simulink model "vtg"  (R2025b)
settings: Solver=FixedStepAuto  StartTime=0.0  StopTime=inf  FixedStep=0.05  RelTol=1e-3
libraries: robotlib x11
settings Model: Creator=sprinkle  LastModifiedBy=sprinkle
settings OptimizationCC: DefaultParameterBehavior=Inlined  EnhancedBackFolding=on  PassReuseOutputArgsAs=Individual arguments  ZeroExternalMemoryAtStartup=off  ZeroInternalMemoryAtStartup=off  MaxStackSize=64  OptimizeBlockOrder=speed  DifferentSizesBufferReuse=on  OptimizationCustomize=off  EfficientTunableParamExpr=on
settings DebuggingCC: ParameterTunabilityLossMsg=error
settings HardwareCC: ProdBitPerPointer=32.0  ProdBitPerSizeT=32.0  ProdBitPerPtrDiffT=32.0  ProdLargestAtomicFloat=None  ProdIntDivRoundTo=Undefined  ProdEndianess=Unspecified  ProdWordSize=32.0  ProdHWDeviceType=Generic->Unspecified (assume 32-bit Generic)
settings SFSimCC: MATLABDynamicMemAlloc=off
settings RTWCC: SystemTargetFile=ert.tlc  HardwareBoard=Robot Operating System (ROS)  TLCOptions="-aInlineSetEventsForThisBaseRateFcn=TLC_FALSE -aSuppressMultiTaskScheduler=TLC_FALSE  -aRateBasedStepFcn=0"  GenCodeOnly=on  TemplateMakefile=ert_default_tmf  Toolchain=Catkin  TargetLang=C++  Description=Embedded Coder
settings CodeAppCC: ForceParamTrailComments=on  IgnoreCustomStorageClasses=off  OperatorAnnotations=on  SimulinkDataObjDesc=on  SFDataObjDesc=on  InsertBlockDesc=on

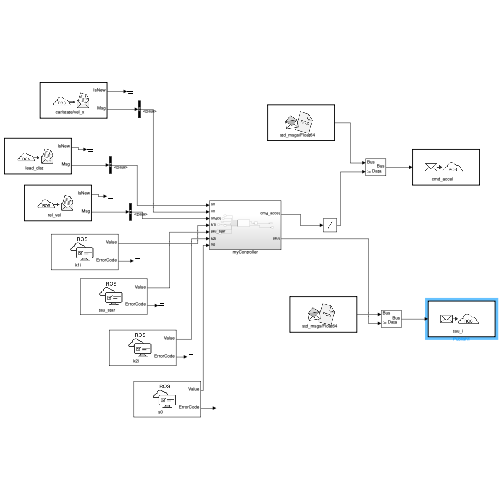
[thumbnail: Simulink's stored preview of the top-level diagram]
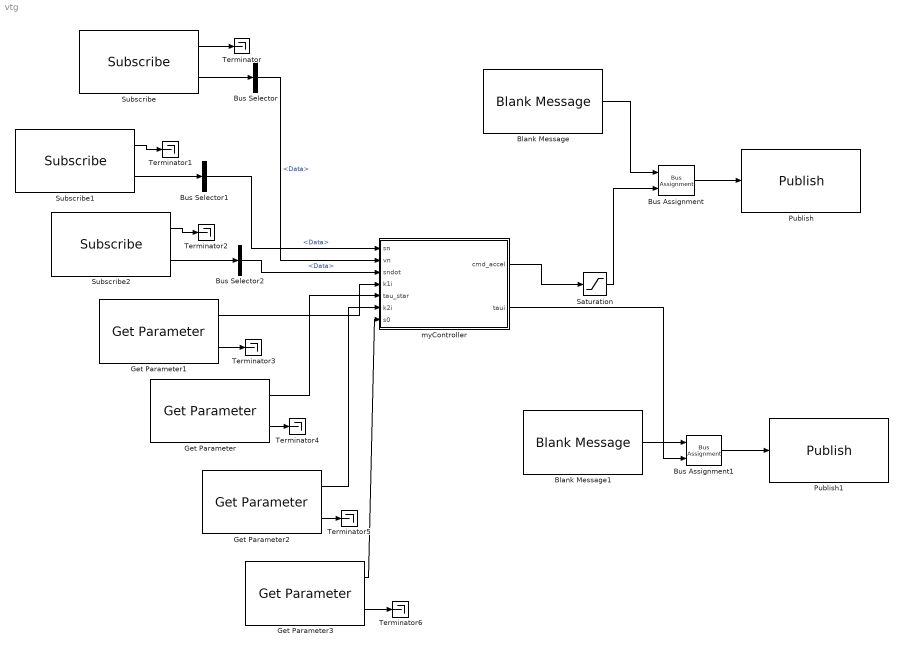
== system vtg ==
  Blank Message : robotlib/Blank Message  messageClass=Message  entityType=std_msgs/Float64  messageType=std_msgs/Float64  SampleTime=inf  legacyBusStruct=off
  Blank Message1 : robotlib/Blank Message  messageClass=Message  entityType=std_msgs/Float64  messageType=std_msgs/Float64  SampleTime=inf  legacyBusStruct=off
  Bus Assignment : BusAssignment  AssignedSignals=Data
  Bus Assignment1 : BusAssignment  AssignedSignals=Data
  Bus Selector : BusSelector  OutputSignals=Data
  Bus Selector1 : BusSelector  OutputSignals=Data
  Bus Selector2 : BusSelector  OutputSignals=Data
  Get Parameter : robotlib/Get Parameter  ParameterSource=Specify your own  ParameterName=tau_star  ParameterType=double  ParameterMaxArrayLength=16  ParameterInitialValue=2.0  SampleTime=-1  ShowErrorCodeOutput=on  ModelName=vtg  BlockId=ParamGet_vtg_18
  Get Parameter1 : robotlib/Get Parameter  ParameterSource=Specify your own  ParameterName=k1i  ParameterType=double  ParameterMaxArrayLength=16  ParameterInitialValue=1.1  SampleTime=-1  ShowErrorCodeOutput=on  ModelName=vtg  BlockId=ParamGet_vtg_19
  Get Parameter2 : robotlib/Get Parameter  ParameterSource=Specify your own  ParameterName=k2i  ParameterType=double  ParameterMaxArrayLength=16  ParameterInitialValue=0.1  SampleTime=-1  ShowErrorCodeOutput=on  ModelName=vtg  BlockId=ParamGet_vtg_52
  Get Parameter3 : robotlib/Get Parameter  ParameterSource=Specify your own  ParameterName=s0  ParameterType=double  ParameterMaxArrayLength=16  ParameterInitialValue=0.1  SampleTime=-1  ShowErrorCodeOutput=on  ModelName=vtg  BlockId=ParamGet_vtg_54
  Publish : robotlib/Publish  topicSource=Specify your own  topic=cmd_accel  messageType=std_msgs/Float64  legacyBusStruct=off  messageQueueLength=1
  Publish1 : robotlib/Publish  topicSource=Specify your own  topic=tau_i  messageType=std_msgs/Float64  legacyBusStruct=off  messageQueueLength=1
  Saturation : Saturate  UpperLimit=1.5  LowerLimit=-3.0
  Subscribe : robotlib/Subscribe  topicSource=Specify your own  topic=car/state/vel_x  messageType=std_msgs/Float64  SampleTime=-1  legacyBusStruct=off  messageQueueLength=1
  Subscribe1 : robotlib/Subscribe  topicSource=Specify your own  topic=lead_dist  messageType=std_msgs/Float64  SampleTime=-1  legacyBusStruct=off  messageQueueLength=1
  Subscribe2 : robotlib/Subscribe  topicSource=Specify your own  topic=rel_vel  messageType=std_msgs/Float64  SampleTime=-1  legacyBusStruct=off  messageQueueLength=1
  Terminator{,1..6} (7 alike) : Terminator
  myController : Subsystem
  wires:
  Subscribe/2 -> Bus Selector/1
  Subscribe/1 -> Terminator/1
  Subscribe1/1 -> Terminator1/1
  Blank Message/1 -> Bus Assignment/1
  Bus Assignment/1 -> Publish/1
  Bus Selector/1 -> myController/2(vn)  "<Data>"
  myController/1(cmd_accel) -> Saturation/1
  Get Parameter/1 -> myController/5(tau_star)
  Get Parameter1/1 -> myController/4(k1i)
  Saturation/1 -> Bus Assignment/2
  Subscribe1/2 -> Bus Selector1/1
  Bus Selector1/1 -> myController/1(sn)  "<Data>"
  Subscribe2/1 -> Terminator2/1
  Bus Selector2/1 -> myController/3(sndot)  "<Data>"
  Subscribe2/2 -> Bus Selector2/1
  Get Parameter1/2 -> Terminator3/1
  Get Parameter/2 -> Terminator4/1
  Get Parameter2/1 -> myController/6(k2i)
  Get Parameter2/2 -> Terminator5/1
  Get Parameter3/2 -> Terminator6/1
  Get Parameter3/1 -> myController/7(s0)
  Bus Assignment1/1 -> Publish1/1
  myController/2(taui) -> Bus Assignment1/2
  Blank Message1/1 -> Bus Assignment1/1

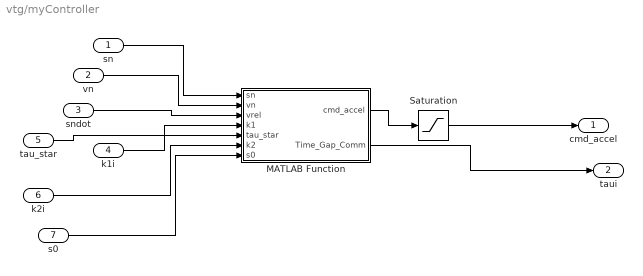
== system vtg/myController ==
  sn : Inport
  vn : Inport  Port=2
  sndot : Inport  Port=3
  k1i : Inport  Port=4
  tau_star : Inport  Port=5
  k2i : Inport  Port=6
  s0 : Inport  Port=7
  MATLAB Function : MATLAB Function  TreatAsAtomicUnit=on
  Saturation : Saturate  UpperLimit=1.5  LowerLimit=-3
  cmd_accel : Outport
  taui : Outport  Port=2
  wires:
  MATLAB Function/1(cmd_accel) -> Saturation/1
  k1i/1 -> MATLAB Function/4(k1)
  sn/1 -> MATLAB Function/1(sn)
  vn/1 -> MATLAB Function/2(vn)
  sndot/1 -> MATLAB Function/3(vrel)
  k2i/1 -> MATLAB Function/6(k2)
  s0/1 -> MATLAB Function/7(s0)
  tau_star/1 -> MATLAB Function/5(tau_star)
  Saturation/1 -> cmd_accel/1
  MATLAB Function/2(Time_Gap_Comm) -> taui/1

== matlab function vtg/myController/MATLAB Function ==
  data: sn input; cmd_accel output; vn input; vrel input; k1 input; tau_star input; k2 input; s0 input; Time_Gap_Comm output
function [cmd_accel, Time_Gap_Comm] = vtg_acc_fcn(sn, vn, vrel, k1, tau_star, k2, s0)

coder.extrinsic('icare'); 

rho_s = 0.2;
rho_v = 0.5;
rho_u = 1.0;
gamma = 0.95;
Asys = [0 -1; k1 (-k1*tau_star-k2)];
Bdist = [1; k2];
Csys = [rho_s 0; 0 rho_v; 0 0];
Ru = rho_u^2;
Rmat = [-1/gamma^2 0; 0 inv(Ru)];

ve = vrel + vn;
s_err = sn - (s0+tau_star*ve);
v_err = vn - ve;
Bctrl = [0; -k1*ve];
P=zeros(2);
% TODO: come up with a code-generatable ricatti equation solution
[P, ~, ~] = icare(Asys, [Bdist, Bctrl], Csys'*Csys, Rmat, [], [], []);

ui = -inv(Ru)*([0 -k1*vn]*P*[s_err; v_err]);
Time_Gap_Comm = max(tau_star + double(ui), 0);
cmd_accel = k1*(sn-s0-Time_Gap_Comm*vn) + k2*vrel;

end
